simulink model "ic_completo_blocos"  (Simulink 7.5)
settings: Solver=ode14x  StartTime=0.0  StopTime=Inf  FixedStep=Ts  RelTol=1e-3
PostLoadFcn:
  | , if any(exist('dsrtsu_mdlpostloadfcn', 'file') == [2, 3, 6]), try dsrtsu_mdlpostloadfcn('Execute', bdroot); catch fprintf('Error in PostLoadFcn (dsrtsu_mdlpostloadfcn) for model "%s":\n %s\n', bdroot, lasterr); end, end,
InitFcn:
  | iC_ini
values from neighbouring files (symbols this model uses):
  C = Cideal+deltaC    (= 4e-05)    [IMC_calculo_limites_thetas.m]    (also in IMC_ini.m; JORGE_controlador_LCL_malha_interna.m; LCL_PAPM.m; R_in_LCL.m)
  L1 = L1ideal+deltaL1    (= 0.002)    [IMC_calculo_limites_thetas.m]    (also in IMC_ini.m; LCL_PAPM.m; R_in_LCL.m; calculo_FTs.m)
  L2 = L2ideal+deltaL2+Lgideal+deltaLg    (= 0.002)    [IMC_calculo_limites_thetas.m]    (also in IMC_ini.m; LCL_PAPM.m; R_in_LCL.m; calculo_FTs.m)
  R1 = R1ideal+deltaR1    (= 1)    [IMC_calculo_limites_thetas.m]    (also in IMC_ini.m; R_in_LCL.m = 0; gera_resultados.m = 0; iC_ini.m = 0)
  R2 = R2ideal+deltaR2+Rgideal+deltaRg    (= 1)    [IMC_calculo_limites_thetas.m]    (also in IMC_ini.m; R_in_LCL.m = 0; gera_resultados.m = 0; iC_ini.m = 0)
  Ts = 0.5    [IMC_calculo_limites_thetas.m]    (also in IMC_datta_ini.m; IMC_ini.m = 8.33333333333e-05; JORGE_controlador_LCL_malha_interna.m = 8.33333333333e-05; LCL_PAPM.m = 8.33333333333e-05)
undefined symbols (not defined in the file or in its folder): MRD, MRN
libraries: powerlib x9, powerlib_extras x1
settings Model: DSRTSU_INTERNAL_RTI_VER=390  DSRTSU_INTERNAL_RTI_TYPE=rti1103  Creator=Marcelo  LastModifiedBy=dpbernardon
settings SolverCC: ExtrapolationOrder=1
settings OptimizationCC: BlockReduction=off  ExpressionDepthLimit=128
settings DebuggingCC: FcnCallInpInsideContextMsg=Enable All
settings HardwareCC: ProdIntDivRoundTo=Zero  ProdEndianess=BigEndian  ProdHWDeviceType=Generic->Custom  TargetIntDivRoundTo=Zero  TargetEndianess=BigEndian  TargetHWDeviceType=Generic->Custom
settings ModelReferenceCC: ModelReferenceMinAlgLoopOccurrences=on
settings RTWCC: SystemTargetFile=rti1103.tlc  MakeCommand=make_rti  TemplateMakefile=rti1103.tmf  Description=dSPACE DS1103 Hardware Platform  ProcessScript=rti1103_make_rtw_hook
settings STFCustomTargetCC: ParMdlRefBuildCompliant=on  GeneratePreprocessorConditionals=Disable all  SystemTargetFile=rti1103.tlc
settings GRTTargetCC: CompOptLevelCompliant=off  MatFileLogging=off  ExtModeMexFile=noextcomm
settings CustomProperty: DataType=RTWOptions_EnumType_C__dSPACE RCPHIL 72_matlab_rti1103_tlc_rti1103_1InitialSimState  Value=RUN
settings EnumStrPairs: String=RUN

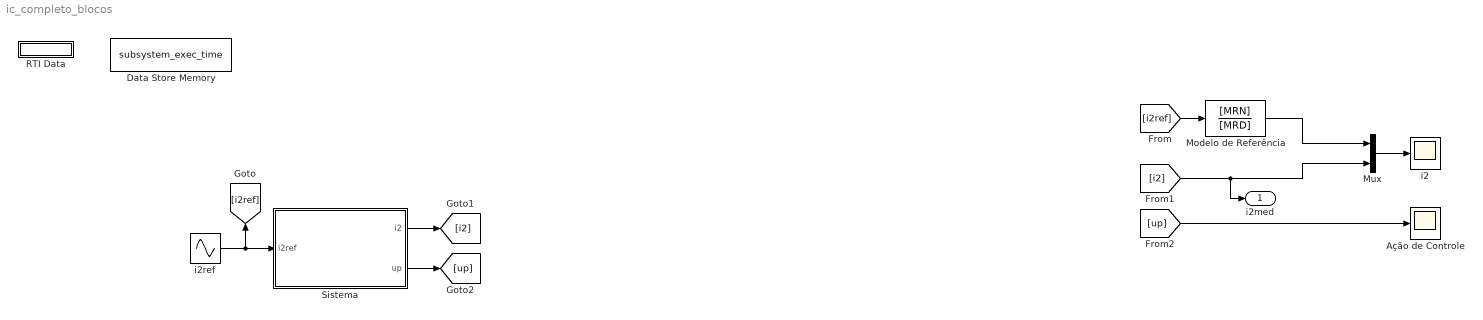
== system ic_completo_blocos ==
  Ação de Controle : Scope
      settings: YMin=-50  YMax=50
  Data Store Memory : DataStoreMemory  DataStoreName=subsystem_exec_time  ReadBeforeWriteMsg=warning  WriteAfterWriteMsg=warning  WriteAfterReadMsg=warning  OutDataType=fixdt(1, 16)  OutScaling=2^0
      settings: RTWStateStorageClass=ExportedGlobal
  Modelo de Referência : DiscreteTransferFcn  Numerator=[MRN]  Denominator=[MRD]  SampleTime=Ts
  Mux : Mux  Inputs=2
  RTI Data : Subsystem  Tag=struct('RTIDataServer',struct('RTIDataServerVs','2','RTIModelDescription','struct(''main'',''ic_completo_blocos'',''sub'','''',''isMp'',0)'))  LoadFcn="if exist('rtidc'), try,  rtidc('DataHostBlockClbLoad', gcbh); catch, disp(['Warning: ''LoadFcn'' for RTI Data block failed: ' lasterr]); end, end,"
      settings: CopyFcn="if exist('rtidc'), try,  rtidc('DataHostBlockClbCopy', gcbh); catch, disp(['Warning: ''CopyFcn'' for RTI Data block failed: ' lasterr]); end, end,"  DeleteFcn="if exist('rtidc'), try,  rtidc('DataHostBlockClbDelete', gcbh); catch, disp(['Warning: ''DeleteFcn'' for RTI Data block failed: ' lasterr]); end, end,"  ModelCloseFcn="if exist('rtidc'), try,  rtidc('DataHostBlockClbModelClose', gcbh); catch, disp(['Warning: ''ModelCloseFcn'' for RTI Data block failed: ' lasterr]); end, end,"  PreSaveFcn="if exist('rtidc'), try,  rtidc('DataHostBlockClbPreSave', gcbh); catch, disp(['Warning: ''PreSaveFcn'' for RTI Data block failed: ' lasterr]); end, end,"  PostSaveFcn="if exist('rtidc'), try,  rtidc('DataHostBlockClbPostSave', gcbh); catch, disp(['Warning: ''PostSaveFcn'' for RTI Data block failed: ' lasterr]); end, end,"  NameChangeFcn="if exist('rtidc'), try,  rtidc('DataHostBlockClbNameChange', gcbh); catch, disp(['Warning: ''NameChangeFcn'' for RTI Data block failed: ' lasterr]); end, end,"
      mask Type: RTI_DATA_HOST
      mask Description:
      | RTI Data Block.
      | This block is used by RTI to store internal model-dependent data.
      | Please keep this block on the root level of the model. Deleting this block will result in data loss.
      | 
      | NEVER DELETE OR COPY THIS BLOCK!
      mask Help:
      | RTI Data Block.
      | This block is used by RTI to store internal model-dependent data.
      | Please keep this block on the root level of the model. Deleting this block will result in data loss.
      | 
      | NEVER DELETE OR COPY THIS BLOCK!
      mask Display:
      | text(0.5, 0.5, 'RTI Data', 'HorizontalAlignment', 'center');
      | plot([1 0]);
  Sistema : Subsystem  TreatAsAtomicUnit=on
  i2 : Scope
      settings: YMin=-50  YMax=50
  i2ref : Sin  Amplitude=2  Bias=0  Frequency=2*pi*60  Phase=0  Samples=10  SampleTime=Ts  Offset=0
  i2med : Outport  OutDataType=fixdt(1, 16)  OutScaling=2^0
  wires:
  Mux/1 -> i2/1
  Modelo de Referência/1 -> Mux/1
  [i2ref] -> Modelo de Referência/1
  [i2] -> Mux/2, i2med/1
  [up] -> Ação de Controle/1
  i2ref/1 -> Sistema/1(i2ref), [i2ref]
  Sistema/1(i2) -> [i2]
  Sistema/2(up) -> [up]

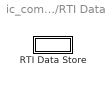
== system ic_completo_blocos/RTI Data ==
  RTI Data Store : Subsystem  Tag="struct('private',struct('version',struct('dsVer',uint32(2),'dsVerCreation',uint32(2),'RTI',struct('ver','6.8','type','RTI1103')),'access',struct('type','Model','isPerm',1,'created',['17-Jul-2013 18:57:58'],'modified',['23-Aug-2013 14:03:43'],'location','')),'public',struct('main',struct('data',[]),'sub',struct('name',{{'ic_completo_blocos'}},'data',{{struct('TH',struct('thTaskInfo',struct('taskType',{'TIMER','HWINT','TMRINT','SWINT'},'tasksNumOf',{1,0,0,0},'srcIds',{{'TIMERA'},{},{},{}},'taskNames',{{['Timer Task 1']},{},{},{}})),'th_tc',struct('dataType','TASK','taskGroupId','','taskGroupList',{{}},'taskSchedulingPolicy','FCFS','taskType','TIMER','blkh',-1,'srcId','TIMERA','srcSgnName',['Timer A interrupt'],'srcCpuName','','taskName',['Timer Task 1  [8.33333e-005] s'],'taskNameDisplayExt','','smplTime',8.3333333333333331e-05,'smplTimeOffs',0,'hasFixedPriority',0,'priority',1,'hasFixedOvc',0,'ovcType',1,'ovcMax',1),'tc_th',struct('dataType','TASK','taskGroupId','','taskGroupList',{{}},'taskSchedulingPolicy','FCFS','taskType','TIMER','blkh',-1,'srcId','TIMERA','srcSgnName',['Timer A interrupt'],'srcCpuName','','taskName',['Timer Task 1  [8.33333e-005] s'],'taskNameDisplayExt','','smplTime',8.3333333333333331e-05,'smplTimeOffs',0,'hasFixedPriority',0,'priority',1,'hasFixedOvc',0,'ovcType',1,'ovcMax',1))}})))"
      mask Type: RTI_DATA_STORE
      mask Description:
      | RTI Data Store Block. This block is used by RTI to store internal model dependent data. Deleting this block will result in data loss.
      | 
      | NEVER DELETE, COPY, OR MODIFY THIS BLOCK!
      mask Help:
      | RTI Data Store Block. This block is used by RTI to store internal model dependent data. Deleting this block will result in data loss.
      | 
      | NEVER DELETE, COPY, OR MODIFY THIS BLOCK!
      mask Display: text(0.5, 0.5, ' ', 'HorizontalAlignment', 'center');

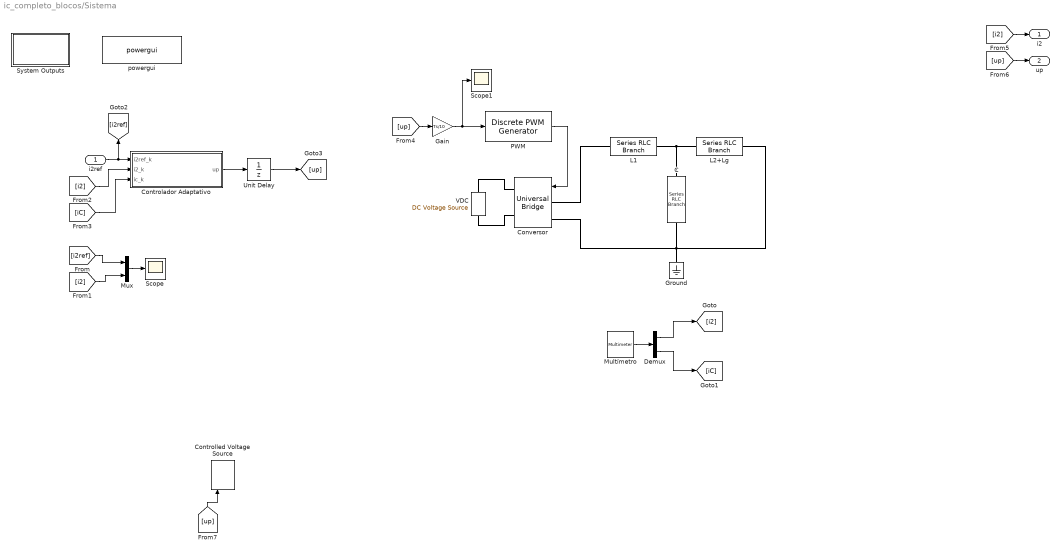
== system ic_completo_blocos/Sistema ==
  i2ref : Inport
  C : powerlib/Elements/Series RLC Branch  DialogController=POWERSYS.PowerSysDialog  PhysicalDomain=powersysdomain  SubClassName=unknown  LeftPortType=p1  RightPortType=p1  LConnTagsString=__new0  RConnTagsString=__new0  BranchType=C  Resistance=1  Inductance=1e-3  SetiL0=off  InitialCurrent=0  Capacitance=C  Setx0=off  InitialVoltage=0  Measurements=Branch current
  Controlador Adaptativo : Stateflow chart  TreatAsAtomicUnit=on  SystemSampleTime=Ts
      settings: MinAlgLoopOccurrences=on  RTWSystemCode=Function
  Controlled Voltage Source : powerlib/Electrical Sources/Controlled Voltage Source  DialogController=POWERSYS.PowerSysDialog  SystemSampleTime=-1  Initialize=on  Source_Type=AC  Amplitude=0  Phase=0  Frequency=0  Measurements=None
  Conversor : powerlib/Power Electronics/Universal Bridge  DialogController=POWERSYS.PowerSysDialog  SystemSampleTime=-1  Arms=2  SnubberResistance=1e5  SnubberCapacitance=inf  Device=IGBT / Diodes  Ron=1e-3  Lon=0  ForwardVoltages="[  0  0  ]"  ForwardVoltage=0  GTOparameters=[ 10e-6 , 20e-6 ]  IGBTparameters=[ 1e-6 , 2e-6 ]  Measurements=None  Measurements_2=None  converterType=Rectifier
  Demux : Demux  Outputs=2
  Gain : Gain  Gain=Ts/10  ParameterDataType=fixdt(1, 16)  ParameterScaling=2^0  OutDataType=fixdt(1, 16)  OutScaling=2^0  SampleTime=Ts
  Ground : powerlib/Elements/Ground  DialogController=POWERSYS.PowerSysDialog  PhysicalDomain=powersysdomain  SubClassName=unknown  LeftPortType=p1  RightPortType=p1  LConnTagsString=a
  L1 : powerlib/Elements/Series RLC Branch  DialogController=POWERSYS.PowerSysDialog  PhysicalDomain=powersysdomain  SubClassName=unknown  LeftPortType=p1  RightPortType=p1  LConnTagsString=__new0  RConnTagsString=__new0  BranchType=RL  Resistance=R1  Inductance=L1  SetiL0=off  InitialCurrent=0  Capacitance=1e-6  Setx0=off  InitialVoltage=0  Measurements=None
  L2+Lg : powerlib/Elements/Series RLC Branch  DialogController=POWERSYS.PowerSysDialog  PhysicalDomain=powersysdomain  SubClassName=unknown  LeftPortType=p1  RightPortType=p1  LConnTagsString=__new0  RConnTagsString=__new0  BranchType=RL  Resistance=R2  Inductance=L2  SetiL0=off  InitialCurrent=0  Capacitance=1e-6  Setx0=off  InitialVoltage=0  Measurements=Branch current
  Multímetro : powerlib/Measurements/Multimeter  SystemSampleTime=-1  PhasorSimulation=off  OutputType=Complex  sel=[2 1]  L=2  Gain=[1 1]  yselected={'Ib: Sistema/L2+Lg','Ib: Sistema/C'};  PSBOutputType=1  PSBequivalent=0  AxesSetting=[0,0.1,-100,100]  Display=0  SavedBlockNames=-11
  Mux : Mux  Inputs=2
  PWM : powerlib_extras/Discrete  Control Blocks/Discrete PWM Generator  DialogController=POWERSYS.PowerSysDialog  SystemSampleTime=-1  GeneratorMode="2-arm  bridge (4 pulses)"  Fc=12000  Ts=Ts  Internal=off  mIndex=0.4  Freq=60  Phase=0
  Scope : Scope
      settings: TimeRange=0.073656578134651  YMin=-3  YMax=3  SaveName=ScopeData2
  Scope1 : Scope
      settings: TimeRange=0.073656578134651  YMin=-3  YMax=3  SaveName=ScopeData3
  System Outputs : Subsystem  mask(System Outputs){ShowInLibBrowser=0}
      mask prompts: ShowInLibBrowser "Mask Parameter 1:"
      mask help: Add code to a systems Outputs function
      settings: CopyFcn=cccopyfcn(gcb)  OpenFcn=ccopenfcn('System Outputs Function')
      mask Help: eval('feval(''rtwprivate'',''rtwhelpview'',''rtw_sys_outputs_block'')');
      mask Display: disp('System\nOutputs');
  Unit Delay : UnitDelay  SampleTime=-1
  VDC : powerlib/Electrical Sources/DC Voltage Source  DialogController=POWERSYS.PowerSysDialog  SystemSampleTime=-1  Amplitude=10  Measurements=None
  powergui : powerlib/powergui  Priority=1  SystemSampleTime=-1  SimulationMode=Discrete  SampleTime=Ts  frequency=60  SPID=off  DisableSnubberDevices=off  DisableRonSwitches=off  DisableVfSwitches=off  SwTol=0  Interpol=off  frequencyindice=0  echomessages=off  HookPort=off  DisplayEquations=off  FunctionMessages=off  EnableUseOfTLC=off  x0status=blocks  RestoreLinks=warning  ResistiveCurrentMeasurement=off  Ylog=off  Xlog=on  ShowGrid=off  save=off  variable=ZData  ZoomFFT=off  StartTime=0.0  cycles=1  DisplayStyle=1  FreqAxis=off  MaxFrequency=1000  frequencyindicesteady=1  display=off  methode=off
  i2 : Outport  OutDataType=fixdt(1, 16)  OutScaling=2^0
  up : Outport  Port=2  OutDataType=fixdt(1, 16)  OutScaling=2^0
  wires:
  i2ref/1 -> Controlador Adaptativo/1(i2ref_k), [i2ref]
  Mux/1 -> Scope/1
  Demux/1 -> [i2]
  Demux/2 -> [iC]
  [i2ref] -> Mux/1
  [i2] -> Controlador Adaptativo/2(i2_k)
  Controlador Adaptativo/1(up) -> Unit Delay/1
  [i2] -> i2/1
  [up] -> up/1
  Multímetro/1 -> Demux/1
  [iC] -> Controlador Adaptativo/3(ic_k)
  [up] -> Controlled Voltage Source/1
  Unit Delay/1 -> [up]
  [i2] -> Mux/2
  [up] -> Gain/1
  Gain/1 -> PWM/1, Scope1/1
  PWM/1 -> Conversor/1
  connections:
  L2+Lg/LConn1 -- L1/RConn1 -- C/LConn1
  L2+Lg/RConn1 -- C/RConn1 -- Ground/LConn1 -- Conversor/LConn2
  Conversor/RConn1 -- VDC/RConn1
  VDC/LConn1 -- Conversor/RConn2
  Conversor/LConn1 -- L1/LConn1

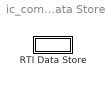
== system ic_completo_blocos/RTI Data/RTI Data Store ==
  RTI Data Store : Subsystem
      mask Type: RTI_DATA_STORE
      mask Description:
      | RTI Data Store Block. This block is used by RTI to store internal model dependent data. Deleting this block will result in data loss.
      | 
      | NEVER DELETE, COPY, OR MODIFY THIS BLOCK!
      mask Help:
      | RTI Data Store Block. This block is used by RTI to store internal model dependent data. Deleting this block will result in data loss.
      | 
      | NEVER DELETE, COPY, OR MODIFY THIS BLOCK!
      mask Display: text(0.5, 0.5, ' ', 'HorizontalAlignment', 'center');

== system ic_completo_blocos/Sistema/System Outputs ==

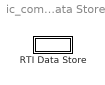
== system ic_completo_blocos/RTI Data/RTI Data Store/RTI Data Store ==
  RTI Data Store : Subsystem
      mask Type: RTI_DATA_STORE
      mask Description:
      | RTI Data Store Block. This block is used by RTI to store internal model dependent data. Deleting this block will result in data loss.
      | 
      | NEVER DELETE, COPY, OR MODIFY THIS BLOCK!
      mask Help:
      | RTI Data Store Block. This block is used by RTI to store internal model dependent data. Deleting this block will result in data loss.
      | 
      | NEVER DELETE, COPY, OR MODIFY THIS BLOCK!
      mask Display: text(0.5, 0.5, ' ', 'HorizontalAlignment', 'center');

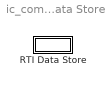
== system ic_completo_blocos/RTI Data/RTI Data Store/RTI Data Store/RTI Data Store ==
  RTI Data Store : Subsystem
      mask Type: RTI_DATA_STORE
      mask Description:
      | RTI Data Store Block. This block is used by RTI to store internal model dependent data. Deleting this block will result in data loss.
      | 
      | NEVER DELETE, COPY, OR MODIFY THIS BLOCK!
      mask Help:
      | RTI Data Store Block. This block is used by RTI to store internal model dependent data. Deleting this block will result in data loss.
      | 
      | NEVER DELETE, COPY, OR MODIFY THIS BLOCK!
      mask Display: text(0.5, 0.5, ' ', 'HorizontalAlignment', 'center');

== system ic_completo_blocos/RTI Data/RTI Data Store/RTI Data Store/RTI Data Store/RTI Data Store ==

== matlab function Sistema/Controlador Adaptativo ==
  data: i2ref_k input double; up output double; i2_k input double; ic_k input double
function up  = adaptativo( i2ref_k, i2_k, ic_k )

%#CODEGEN

%Definição dos valores projetados dos elementos do filtro
L1ideal=5e-3;
L2ideal=5e-3;
Lgideal=0;
Cideal=40e-6;
R1ideal=0;
R2ideal=0;
Rgideal=0;

%Definição de erros percentuais para simular variação paramétrica
errL1=0;
errL2=0;
errLg=0;
errC=0;
errR1=0;
errR2=0;
errRg=0;
deltaL1=errL1*L1ideal;
deltaL2=errL2*L2ideal;
deltaLg=errLg*Lgideal;
deltaC=errC*Cideal;
deltaR1=errR1*R1ideal;
deltaR2=errR2*R2ideal;
deltaRg=errRg*Rgideal;

%Definição do valor real medido, incluindo a variação paramétrica
%percentual
L1=L1ideal+deltaL1;
L2=L2ideal+deltaL2+Lgideal+deltaLg;
C=Cideal+deltaC;
R1=R1ideal+deltaR1;
R2=R2ideal+deltaR2+Rgideal+deltaRg;

%Demais elementos
Ts=1/12000;
w=sqrt((L1+L2)/(L1*L2*C));

%Kp é a multiplicação do ganho do controlador da malha interna(kp), do
%ganho da planta(ki) e do ganho da malha externa(kod)
kp=50;
ki=sin(w*Ts)/(w*L1);
kod=Ts^2/(C*L2);
Kp=kp*ki*kod;

%polos do modelo de referência:
p1=0.1;
p2=0.1;
p3=0.1;

km=(1-p1)*(1-p2)*(1-p3);

%constantes -> gamaD < (1-gama)*km/kp
gamaD=km/kp - 2e-3;
gama=1e-3;

%% Variáveis Persistentes e Inicializações

persistent theta_k;
if isempty(theta_k)
    theta_k=[-0.4716; -0.3125; 0.1089; 0.006822; -0.252; -0.1836; -0.4857; 0.8682];
%    theta_k(1)=0; %theta11_k \
%    theta_k(2)=0; %theta12_k  | theta1
%    theta_k(3)=0; %theta13_k /
%    theta_k(4)=0; %theta21_k \
%    theta_k(5)=0; %theta22_k  | theta2
%    theta_k(6)=0; %theta23_k /
%    theta_k(7)=0; %theta3_k > theta3
%    theta_k(8)=0;%theta4_k > thata4
end

persistent omega_k;
if isempty(omega_k)
    omega_k=[0; 0; 0; 0; 0; 0; 0; 0];
%    omega_k(1)=0; %u_k-1 \
%    omega_k(2)=0; %u_k-2 | w1
%    omega_k(3)=0; %u_k-3 /
%    omega_k(4)=0; %i2_k-1 \
%    omega_k(5)=0; %i2_k-2 | w2
%    omega_k(6)=0; %i2_k-3 /
%    omega_k(7)=0; %i2_k
%    omega_k(8)=0;%i2ref_k
end

persistent omega_k_1;
if isempty(omega_k_1)
    omega_k_1=[0; 0; 0; 0; 0; 0; 0; 0];
end

persistent omega_k_2;
if isempty(omega_k_2)
    omega_k_2=[0; 0; 0; 0; 0; 0; 0; 0];
end

persistent omega_k_3;
if isempty(omega_k_3)
    omega_k_3=[0; 0; 0; 0; 0; 0; 0; 0];
end

persistent eta_k_1;
if isempty(eta_k_1)
    eta_k_1=[0; 0; 0; 0; 0; 0; 0; 0];
end

persistent eta_k_2;
if isempty(eta_k_2)
    eta_k_2=[0; 0; 0; 0; 0; 0; 0; 0];
end

persistent eta_k_3;
if isempty(eta_k_3)
    eta_k_3=[0; 0; 0; 0; 0; 0; 0; 0];
end

persistent i2m_k_1;
if isempty(i2m_k_1)
    i2m_k_1=0;
end

persistent i2m_k_2;
if isempty(i2m_k_2)
    i2m_k_2=0;
end

persistent i2m_k_3;
if isempty(i2m_k_3)
    i2m_k_3=0;
end

persistent i2ref_k_1;
if isempty(i2ref_k_1)
    i2ref_k_1=0;
end

persistent i2ref_k_2;
if isempty(i2ref_k_2)
    i2ref_k_2=0;
end

persistent i2ref_k_3;
if isempty(i2ref_k_3)
    i2ref_k_3=0;
end

persistent v_k_1;
if isempty(v_k_1)
    v_k_1=0;
end

persistent v_k_2;
if isempty(v_k_2)
    v_k_2=0;
end

persistent v_k_3;
if isempty(v_k_3)
    v_k_3=0;
end

persistent rho_k;
if isempty(rho_k)
    rho_k=Kp/km;
end


%% Cálculos

%Ação de controle
omega_k(7)= i2_k;
omega_k(8)= i2ref_k;

u_k= theta_k'*omega_k;

%inserindo o controlador proporcional no bloco do adaptativo
up= kp*(u_k-ic_k);

eta_k= (p1+p2+p3)*eta_k_1 - (p1*p2+p1*p3+p2*p3)*eta_k_2 + p1*p2*p3*eta_k_3 + (1-p1)*(1-p2)*(1-p3)*omega_k_3;

i2m_k= (p1+p2+p3)*i2m_k_1 - (p1*p2+p1*p3+p2*p3)*i2m_k_2 + p1*p2*p3*i2m_k_3 + (1-p1)*(1-p2)*(1-p3)*i2ref_k_3;

e1_k= i2_k - i2m_k;
                                                                                          %omega_k(3)=u_k_3
v_k= -(p1+p2+p3)*v_k_1 + (p1*p2+p1*p3+p2*p3)*v_k_2 - p1*p2*p3*v_k_3 - (1-p1)*(1-p2)*(1-p3)*omega_k(3);

q_k= theta_k'*eta_k;

e2_k= v_k+q_k;

ea_k= e1_k+rho_k*e2_k;

m2_k= eta_k'*eta_k + e2_k^2 +1;

%% Atualização

%calcula theta(k+1)
theta_k = theta_k - (gamaD*ea_k/m2_k)*eta_k;

%calcula rho(k+1)
rho_k= rho_k - (gama*ea_k*e2_k)/m2_k;

omega_k_3=omega_k_2;
omega_k_2=omega_k_1;
omega_k_1=omega_k;

omega_k(3)=omega_k(2);
omega_k(2)=omega_k(1);
omega_k(1)=u_k;

omega_k(6)=omega_k(5);
omega_k(5)=omega_k(4);
omega_k(4)=i2_k;

eta_k_3=eta_k_2;
eta_k_2=eta_k_1;
eta_k_1=eta_k;

i2ref_k_3 = i2ref_k_2;
i2ref_k_2 = i2ref_k_1;
i2ref_k_1 = i2ref_k;

i2m_k_3=i2m_k_2;
i2m_k_2=i2m_k_1;
i2m_k_1=i2m_k;

v_k_3=v_k_2;
v_k_2=v_k_1;
v_k_1=v_k;

end
